simulink model "mdaqdemo_enc"  (R2013a)
settings: Solver=FixedStepDiscrete  StartTime=0.0  StopTime=inf  FixedStep=0.01  RelTol=1e-3
libraries: microdaq_lib x4, simulink x2
settings Model: SimulationMode=external  Creator=skibool  LastModifiedBy=witczenko
settings DataIOCC: SignalLoggingSaveFormat=ModelDataLogs
settings OptimizationCC: OptimizeModelRefInitCode=on  LifeSpan=1
settings DebuggingCC: MultiTaskDSMMsg=warning  MultiTaskCondExecSysMsg=none  FrameProcessingCompatibilityMsg=error  StateNameClashWarn=none  StrictBusMsg=None
settings HardwareCC: ProdBitPerLong=40  ProdLargestAtomicInteger=Integer  ProdIntDivRoundTo=Zero  ProdEndianess=LittleEndian  ProdHWDeviceType=Texas Instruments->C6000
settings SFSimCC: SimParseCustomCode=off
settings RTWCC: SystemTargetFile=microdaq.tlc  TemplateMakefile=microdaq.tmf  PostCodeGenCommand=microdaq_postcodegen(buildInfo)  Description=MicroDAQ Real-Time Measurement System
settings CodeAppCC: IgnoreCustomStorageClasses=off
settings STFCustomTargetCC: CodeReplacementLibrary=C89/C90 (ANSI)  CombineOutputUpdateFcns=on  ERTCustomFileBanners=on  SupportContinuousTime=off  SupportNonInlinedSFcns=off  MATLABClassNameForMDSCustomization=Simulink.SoftwareTarget.ERTCustomization  SystemTargetFile=microdaq.tlc
settings ERTTargetCC: CodeReplacementLibrary=C89/C90 (ANSI)  GenerateSampleERTMain=off  ParMdlRefBuildCompliant=off  CompOptLevelCompliant=off  ConcurrentExecutionCompliant=off  ERTFirstTimeCompliant=off  ModelStepFunctionPrototypeControlCompliant=off  CPPClassGenCompliant=off  ExtMode=on  ExtModeStaticAlloc=on  ExtModeMexArgs=getpref('microdaq','TargetIP') 1 4344  InlinedParameterPlacement=Hierarchical  ERTCustomFileTemplate=microdaq_main.tlc

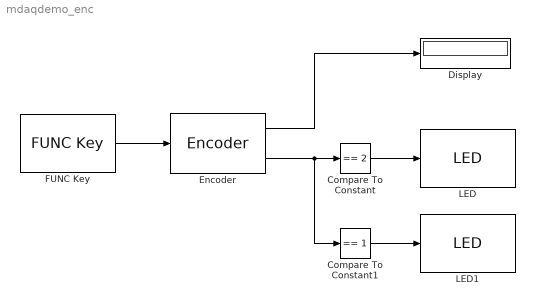
== system mdaqdemo_enc ==
  Compare To Constant : simulink/Logic and Bit Operations/Compare To Constant  relop===  const=2  OutDataTypeStr=uint8
  Compare To Constant1 : simulink/Logic and Bit Operations/Compare To Constant  relop===  const=1  OutDataTypeStr=uint8
  Display : Display
  Encoder : microdaq_lib/Motor Control/Encoder  pChannel=ENC1  SampleTime=0
  FUNC Key : microdaq_lib/Utilities/FUNC Key  pDIOFuncKey=F1  SampleTime=-1
  LED : microdaq_lib/Utilities/LED  SParameter1=D1
  LED1 : microdaq_lib/Utilities/LED  SParameter1=D2
  wires:
  Encoder/1 -> Display/1
  Encoder/2 -> Compare To Constant1/1, Compare To Constant/1
  Compare To Constant/1 -> LED/1
  Compare To Constant1/1 -> LED1/1
  FUNC Key/1 -> Encoder/1
